simulink model "momentumBasedYoga"  (Simulink 9.0)
settings: Solver=FixedStepDiscrete  StartTime=0.0  StopTime="Config.SIMULATION_TIME "  FixedStep=Config.T_STEP  RelTol=1e-3  EnableMultiTasking=on
InitFcn:
  | cd(fileparts(which(bdroot)));
  | initMomentumBasedYoga;
StopFcn:
  | cd(fileparts(which(bdroot)));
  | stopMomentumBasedYoga;
undefined symbols (not defined in the file or in its folder): bVectorConstraints, Config, ConstraintsMatrix, Gain, Reg, ROBOT_DOF, ROBOT_DOF_FOR_SIMULINK, Sat, Sm
libraries: WBToolboxLibrary x80, simulink x4
(part 2 of 2)

== system momentumBasedYoga/Robot State and References/State Machine Yoga/Compute base to fixed link transform ==
  s : Inport
  inertial : Inport  Port=2
  Constant7 : Constant  Value=eye(4)
  "Floating Base to Fixed Link Transform (Left Foot) " : Subsystem
  Floating Base to Fixed Link Transform (Right Foot) : Subsystem
  LFoot to World Transform with Fixed Base : WBToolboxLibrary/wholeBodyModel/Kinematics/Forward Kinematics  frameName=Frames.LEFT_FOOT
      settings: SourceProductName=Whole Body Toolbox
  RFoot to World Transform with Fixed Base : WBToolboxLibrary/wholeBodyModel/Kinematics/Forward Kinematics  frameName=Frames.RIGHT_FOOT
      settings: SourceProductName=Whole Body Toolbox
  fixed_LFoot_H_b : Outport
  fixed_RFoot_H_b : Outport  Port=2
  wires:
  Constant7/1 -> RFoot to World Transform with Fixed Base/1, LFoot to World Transform with Fixed Base/1
  s/1 -> "Floating Base to Fixed Link Transform (Left Foot) "/1(s), Floating Base to Fixed Link Transform (Right Foot)/1(s), LFoot to World Transform with Fixed Base/2, RFoot to World Transform with Fixed Base/2
  "Floating Base to Fixed Link Transform (Left Foot) "/1(fixed_link_H_b) -> fixed_LFoot_H_b/1
  Floating Base to Fixed Link Transform (Right Foot)/1(fixed_link_H_b) -> fixed_RFoot_H_b/1
  RFoot to World Transform with Fixed Base/1 -> Floating Base to Fixed Link Transform (Right Foot)/3(w_H_fixed_link)
  LFoot to World Transform with Fixed Base/1 -> "Floating Base to Fixed Link Transform (Left Foot) "/3(w_H_fixed_link)
  inertial/1 -> "Floating Base to Fixed Link Transform (Left Foot) "/2(inertial), Floating Base to Fixed Link Transform (Right Foot)/2(inertial)

== system momentumBasedYoga/Robot State and References/State Machine Yoga/xCom ==
  w_H_b : Inport
  s : Inport  Port=2
  CoM : WBToolboxLibrary/wholeBodyModel/Kinematics/Forward Kinematics  frameName=Frames.COM
      settings: SourceProductName=Whole Body Toolbox
  "CoM6D ->  CoMXYZ2" : Selector  NumberOfDimensions=2  InputPortWidth=7  IndexOptions=Index vector (dialog),Index vector (dialog)  Indices=[1 2 3],[4]  OutputSizes=1,1
  x_CoM : Outport
  wires:
  s/1 -> CoM/2
  "CoM6D ->  CoMXYZ2"/1 -> x_CoM/1
  CoM/1 -> "CoM6D ->  CoMXYZ2"/1
  w_H_b/1 -> CoM/1

== system momentumBasedYoga/Robot State and References/State Machine Yoga/xCom1 ==
  w_H_b : Inport
  s : Inport  Port=2
  CoM : WBToolboxLibrary/wholeBodyModel/Kinematics/Forward Kinematics  frameName=Frames.COM
      settings: SourceProductName=Whole Body Toolbox
  "CoM6D ->  CoMXYZ2" : Selector  NumberOfDimensions=2  InputPortWidth=7  IndexOptions=Index vector (dialog),Index vector (dialog)  Indices=[1 2 3],[4]  OutputSizes=1,1
  x_CoM : Outport
  wires:
  s/1 -> CoM/2
  "CoM6D ->  CoMXYZ2"/1 -> x_CoM/1
  CoM/1 -> "CoM6D ->  CoMXYZ2"/1
  w_H_b/1 -> CoM/1

== system momentumBasedYoga/Balancing Controller QP/Approximate Momentum Integral/Compute base to fixed link transform/Floating Base to Fixed Link Transform (Left Foot)  ==
  s : Inport
  inertial : Inport  Port=2
  w_H_fixed_link : Inport  Port=3
  Constant : Constant  Value=eye(4)
  Imu to World Transform : WBToolboxLibrary/wholeBodyModel/Kinematics/Forward Kinematics  frameName=Frames.IMU
      settings: SourceProductName=Whole Body Toolbox
  Inv\* : Product  Inputs=/*  Multiplication=Matrix(*)
  "Inv\\*  " : Product  Inputs=/  Multiplication=Matrix(*)
  Neck Position : WBToolboxLibrary/Utilities/Yarp Read  portName=Ports.NECK_POS  signalSize=6  timeout=0.5  blocking=off  timestamp=off  autoconnect=on  errorOnConnection=off
      settings: SourceProductName=Whole Body Toolbox
  Neck Transform : Subsystem
  Switch6 : Switch  Criteria=u2 > Threshold
  USE_IMU4EST_BASE : Constant  Value=Config.USE_IMU4EST_BASE
  fromImuToHomogeousTransformFCN : MATLAB Function  TreatAsAtomicUnit=on
  holder 1 : WBToolboxLibrary/Utilities/holder 
      settings: SourceProductName=Whole Body Toolbox
  holder 2 : WBToolboxLibrary/Utilities/holder 
      settings: SourceProductName=Whole Body Toolbox
  fixed_link_H_b : Outport
  wires:
  Switch6/1 -> fixed_link_H_b/1
  "Inv\\*  "/1 -> fromImuToHomogeousTransformFCN/3(link_H_base), Switch6/3  "link_H_root"
  USE_IMU4EST_BASE/1 -> Switch6/2
  Inv\*/1 -> fromImuToHomogeousTransformFCN/1(imu_H_link), holder 1/1  "imu_H_link"
  holder 2/1 -> fromImuToHomogeousTransformFCN/4(inertial_0)
  Imu to World Transform/1 -> Inv\*/1
  holder 1/1 -> fromImuToHomogeousTransformFCN/2(imu_H_link_0)
  s/1 -> Imu to World Transform/2
  fromImuToHomogeousTransformFCN/1(w_H_b) -> Switch6/1
  inertial/1 -> holder 2/1, fromImuToHomogeousTransformFCN/5(inertial)
  Neck Position/1 -> Neck Transform/1(neck_port)
  Neck Transform/1(neck_pos) -> fromImuToHomogeousTransformFCN/6(neck_pos)
  w_H_fixed_link/1 -> "Inv\\*  "/1, Inv\*/2
  Constant/1 -> Imu to World Transform/1

== system momentumBasedYoga/Balancing Controller QP/Approximate Momentum Integral/Compute base to fixed link transform/Floating Base to Fixed Link Transform (Right Foot) ==
  s : Inport
  inertial : Inport  Port=2
  w_H_fixed_link : Inport  Port=3
  Constant : Constant  Value=eye(4)
  Imu to World Transform : WBToolboxLibrary/wholeBodyModel/Kinematics/Forward Kinematics  frameName=Frames.IMU
      settings: SourceProductName=Whole Body Toolbox
  Inv\* : Product  Inputs=/*  Multiplication=Matrix(*)
  "Inv\\*  " : Product  Inputs=/  Multiplication=Matrix(*)
  Neck Position : WBToolboxLibrary/Utilities/Yarp Read  portName=Ports.NECK_POS  signalSize=6  timeout=0.5  blocking=off  timestamp=off  autoconnect=on  errorOnConnection=off
      settings: SourceProductName=Whole Body Toolbox
  Neck Transform : Subsystem
  Switch6 : Switch  Criteria=u2 > Threshold
  USE_IMU4EST_BASE : Constant  Value=Config.USE_IMU4EST_BASE
  fromImuToHomogeousTransformFCN : MATLAB Function  TreatAsAtomicUnit=on
  holder 1 : WBToolboxLibrary/Utilities/holder 
      settings: SourceProductName=Whole Body Toolbox
  holder 2 : WBToolboxLibrary/Utilities/holder 
      settings: SourceProductName=Whole Body Toolbox
  fixed_link_H_b : Outport
  wires:
  Switch6/1 -> fixed_link_H_b/1
  "Inv\\*  "/1 -> fromImuToHomogeousTransformFCN/3(link_H_base), Switch6/3  "link_H_root"
  USE_IMU4EST_BASE/1 -> Switch6/2
  Inv\*/1 -> fromImuToHomogeousTransformFCN/1(imu_H_link), holder 1/1  "imu_H_link"
  holder 2/1 -> fromImuToHomogeousTransformFCN/4(inertial_0)
  Imu to World Transform/1 -> Inv\*/1
  holder 1/1 -> fromImuToHomogeousTransformFCN/2(imu_H_link_0)
  s/1 -> Imu to World Transform/2
  fromImuToHomogeousTransformFCN/1(w_H_b) -> Switch6/1
  inertial/1 -> holder 2/1, fromImuToHomogeousTransformFCN/5(inertial)
  Neck Position/1 -> Neck Transform/1(neck_port)
  Neck Transform/1(neck_pos) -> fromImuToHomogeousTransformFCN/6(neck_pos)
  w_H_fixed_link/1 -> "Inv\\*  "/1, Inv\*/2
  Constant/1 -> Imu to World Transform/1

== system momentumBasedYoga/Robot State and References/Internal Coordinator/Base to Fixed Link/Fixed Link to World Transform ==
  s : Inport
  Constant1 : Constant  Value=Config.LEFT_RIGHT_FOOT_IN_CONTACT(1)
  Constant7 : Constant  Value=eye(4)
  LFoot to World Transform with Fixed Base = World : WBToolboxLibrary/wholeBodyModel/Kinematics/Forward Kinematics  frameName=Frames.LEFT_FOOT
      settings: SourceProductName=Whole Body Toolbox
  RFoot to World Transform with Fixed Base = World : WBToolboxLibrary/wholeBodyModel/Kinematics/Forward Kinematics  frameName=Frames.RIGHT_FOOT
      settings: SourceProductName=Whole Body Toolbox
  Switch : Switch  Criteria=u2 > Threshold
  w_H_fixed_link : Outport
  wires:
  s/1 -> LFoot to World Transform with Fixed Base = World/2, RFoot to World Transform with Fixed Base = World/2
  Constant7/1 -> RFoot to World Transform with Fixed Base = World/1, LFoot to World Transform with Fixed Base = World/1
  Switch/1 -> w_H_fixed_link/1
  LFoot to World Transform with Fixed Base = World/1 -> Switch/1
  RFoot to World Transform with Fixed Base = World/1 -> Switch/3
  Constant1/1 -> Switch/2

== system momentumBasedYoga/Robot State and References/Internal Coordinator/Base to Fixed Link/Floating Base to Fixed Link Transform  ==
  s : Inport
  inertial : Inport  Port=2
  w_H_fixed_link : Inport  Port=3
  Constant : Constant  Value=eye(4)
  Imu to World Transform : WBToolboxLibrary/wholeBodyModel/Kinematics/Forward Kinematics  frameName=Frames.IMU
      settings: SourceProductName=Whole Body Toolbox
  Inv\* : Product  Inputs=/*  Multiplication=Matrix(*)
  "Inv\\*  " : Product  Inputs=/  Multiplication=Matrix(*)
  Neck Position : WBToolboxLibrary/Utilities/Yarp Read  portName=Ports.NECK_POS  signalSize=6  timeout=0.5  blocking=off  timestamp=off  autoconnect=on  errorOnConnection=off
      settings: SourceProductName=Whole Body Toolbox
  Neck Transform : Subsystem
  Switch6 : Switch  Criteria=u2 > Threshold
  USE_IMU4EST_BASE : Constant  Value=Config.USE_IMU4EST_BASE
  fromImuToHomogeousTransformFCN : MATLAB Function  TreatAsAtomicUnit=on
  holder 1 : WBToolboxLibrary/Utilities/holder 
      settings: SourceProductName=Whole Body Toolbox
  holder 2 : WBToolboxLibrary/Utilities/holder 
      settings: SourceProductName=Whole Body Toolbox
  fixed_link_H_b : Outport
  wires:
  Switch6/1 -> fixed_link_H_b/1
  "Inv\\*  "/1 -> fromImuToHomogeousTransformFCN/3(link_H_base), Switch6/3  "link_H_root"
  USE_IMU4EST_BASE/1 -> Switch6/2
  Inv\*/1 -> fromImuToHomogeousTransformFCN/1(imu_H_link), holder 1/1  "imu_H_link"
  holder 2/1 -> fromImuToHomogeousTransformFCN/4(inertial_0)
  Imu to World Transform/1 -> Inv\*/1
  holder 1/1 -> fromImuToHomogeousTransformFCN/2(imu_H_link_0)
  s/1 -> Imu to World Transform/2
  fromImuToHomogeousTransformFCN/1(w_H_b) -> Switch6/1
  inertial/1 -> holder 2/1, fromImuToHomogeousTransformFCN/5(inertial)
  Neck Position/1 -> Neck Transform/1(neck_port)
  Neck Transform/1(neck_pos) -> fromImuToHomogeousTransformFCN/6(neck_pos)
  w_H_fixed_link/1 -> "Inv\\*  "/1, Inv\*/2
  Constant/1 -> Imu to World Transform/1

== system momentumBasedYoga/Robot State and References/Internal Coordinator/Compute State Velocity/Feet Jacobians ==
  s : Inport
  w_H_b : Inport  Port=2
  Jacobian LFoot : WBToolboxLibrary/wholeBodyModel/Jacobians/Jacobian  frameName=Frames.LEFT_FOOT
      settings: SourceProductName=Whole Body Toolbox
  Jacobian RFoot : WBToolboxLibrary/wholeBodyModel/Jacobians/Jacobian  frameName=Frames.RIGHT_FOOT
      settings: SourceProductName=Whole Body Toolbox
  J_LFoot : Outport
  J_RFoot : Outport  Port=2
  wires:
  Jacobian LFoot/1 -> J_LFoot/1
  Jacobian RFoot/1 -> J_RFoot/1
  w_H_b/1 -> Jacobian RFoot/1, Jacobian LFoot/1
  s/1 -> Jacobian LFoot/2, Jacobian RFoot/2

== system momentumBasedYoga/Robot State and References/State Machine Yoga/Compute State Velocity/Feet Jacobians ==
  s : Inport
  w_H_b : Inport  Port=2
  Jacobian LFoot : WBToolboxLibrary/wholeBodyModel/Jacobians/Jacobian  frameName=Frames.LEFT_FOOT
      settings: SourceProductName=Whole Body Toolbox
  Jacobian RFoot : WBToolboxLibrary/wholeBodyModel/Jacobians/Jacobian  frameName=Frames.RIGHT_FOOT
      settings: SourceProductName=Whole Body Toolbox
  J_LFoot : Outport
  J_RFoot : Outport  Port=2
  wires:
  Jacobian LFoot/1 -> J_LFoot/1
  Jacobian RFoot/1 -> J_RFoot/1
  w_H_b/1 -> Jacobian RFoot/1, Jacobian LFoot/1
  s/1 -> Jacobian LFoot/2, Jacobian RFoot/2

== system momentumBasedYoga/Robot State and References/State Machine Yoga/Compute base to fixed link transform/Floating Base to Fixed Link Transform (Left Foot)  ==
  s : Inport
  inertial : Inport  Port=2
  w_H_fixed_link : Inport  Port=3
  Constant : Constant  Value=eye(4)
  Imu to World Transform : WBToolboxLibrary/wholeBodyModel/Kinematics/Forward Kinematics  frameName=Frames.IMU
      settings: SourceProductName=Whole Body Toolbox
  Inv\* : Product  Inputs=/*  Multiplication=Matrix(*)
  "Inv\\*  " : Product  Inputs=/  Multiplication=Matrix(*)
  Neck Position : WBToolboxLibrary/Utilities/Yarp Read  portName=Ports.NECK_POS  signalSize=6  timeout=0.5  blocking=off  timestamp=off  autoconnect=on  errorOnConnection=off
      settings: SourceProductName=Whole Body Toolbox
  Neck Transform : Subsystem
  Switch6 : Switch  Criteria=u2 > Threshold
  USE_IMU4EST_BASE : Constant  Value=Config.USE_IMU4EST_BASE
  fromImuToHomogeousTransformFCN : MATLAB Function  TreatAsAtomicUnit=on
  holder 1 : WBToolboxLibrary/Utilities/holder 
      settings: SourceProductName=Whole Body Toolbox
  holder 2 : WBToolboxLibrary/Utilities/holder 
      settings: SourceProductName=Whole Body Toolbox
  fixed_link_H_b : Outport
  wires:
  Switch6/1 -> fixed_link_H_b/1
  "Inv\\*  "/1 -> fromImuToHomogeousTransformFCN/3(link_H_base), Switch6/3  "link_H_root"
  USE_IMU4EST_BASE/1 -> Switch6/2
  Inv\*/1 -> fromImuToHomogeousTransformFCN/1(imu_H_link), holder 1/1  "imu_H_link"
  holder 2/1 -> fromImuToHomogeousTransformFCN/4(inertial_0)
  Imu to World Transform/1 -> Inv\*/1
  holder 1/1 -> fromImuToHomogeousTransformFCN/2(imu_H_link_0)
  s/1 -> Imu to World Transform/2
  fromImuToHomogeousTransformFCN/1(w_H_b) -> Switch6/1
  inertial/1 -> holder 2/1, fromImuToHomogeousTransformFCN/5(inertial)
  Neck Position/1 -> Neck Transform/1(neck_port)
  Neck Transform/1(neck_pos) -> fromImuToHomogeousTransformFCN/6(neck_pos)
  w_H_fixed_link/1 -> "Inv\\*  "/1, Inv\*/2
  Constant/1 -> Imu to World Transform/1

== system momentumBasedYoga/Robot State and References/State Machine Yoga/Compute base to fixed link transform/Floating Base to Fixed Link Transform (Right Foot) ==
  s : Inport
  inertial : Inport  Port=2
  w_H_fixed_link : Inport  Port=3
  Constant : Constant  Value=eye(4)
  Imu to World Transform : WBToolboxLibrary/wholeBodyModel/Kinematics/Forward Kinematics  frameName=Frames.IMU
      settings: SourceProductName=Whole Body Toolbox
  Inv\* : Product  Inputs=/*  Multiplication=Matrix(*)
  "Inv\\*  " : Product  Inputs=/  Multiplication=Matrix(*)
  Neck Position : WBToolboxLibrary/Utilities/Yarp Read  portName=Ports.NECK_POS  signalSize=6  timeout=0.5  blocking=off  timestamp=off  autoconnect=on  errorOnConnection=off
      settings: SourceProductName=Whole Body Toolbox
  Neck Transform : Subsystem
  Switch6 : Switch  Criteria=u2 > Threshold
  USE_IMU4EST_BASE : Constant  Value=Config.USE_IMU4EST_BASE
  fromImuToHomogeousTransformFCN : MATLAB Function  TreatAsAtomicUnit=on
  holder 1 : WBToolboxLibrary/Utilities/holder 
      settings: SourceProductName=Whole Body Toolbox
  holder 2 : WBToolboxLibrary/Utilities/holder 
      settings: SourceProductName=Whole Body Toolbox
  fixed_link_H_b : Outport
  wires:
  Switch6/1 -> fixed_link_H_b/1
  "Inv\\*  "/1 -> fromImuToHomogeousTransformFCN/3(link_H_base), Switch6/3  "link_H_root"
  USE_IMU4EST_BASE/1 -> Switch6/2
  Inv\*/1 -> fromImuToHomogeousTransformFCN/1(imu_H_link), holder 1/1  "imu_H_link"
  holder 2/1 -> fromImuToHomogeousTransformFCN/4(inertial_0)
  Imu to World Transform/1 -> Inv\*/1
  holder 1/1 -> fromImuToHomogeousTransformFCN/2(imu_H_link_0)
  s/1 -> Imu to World Transform/2
  fromImuToHomogeousTransformFCN/1(w_H_b) -> Switch6/1
  inertial/1 -> holder 2/1, fromImuToHomogeousTransformFCN/5(inertial)
  Neck Position/1 -> Neck Transform/1(neck_port)
  Neck Transform/1(neck_pos) -> fromImuToHomogeousTransformFCN/6(neck_pos)
  w_H_fixed_link/1 -> "Inv\\*  "/1, Inv\*/2
  Constant/1 -> Imu to World Transform/1

== system momentumBasedYoga/Balancing Controller QP/Approximate Momentum Integral/Compute base to fixed link transform/Floating Base to Fixed Link Transform (Left Foot) /Neck Transform ==
  neck_port : Inport
  Constant : Constant  Value=zeros(3,1)
  Gain : Gain  Gain=pi/180
  Selector1 : Selector  InputPortWidth=6  IndexOptions=Index vector (dialog)  Indices=[1:3]  OutputSizes=1
  Switch : Switch  Criteria=u2 > Threshold
  USE_IMU4EST_BASE1 : Constant  Value=Config.CORRECT_NECK_IMU
  neck_pos : Outport
  wires:
  neck_port/1 -> Gain/1
  USE_IMU4EST_BASE1/1 -> Switch/2
  Switch/1 -> neck_pos/1
  Gain/1 -> Selector1/1
  Constant/1 -> Switch/3
  Selector1/1 -> Switch/1  "neck pos"

== system momentumBasedYoga/Balancing Controller QP/Approximate Momentum Integral/Compute base to fixed link transform/Floating Base to Fixed Link Transform (Right Foot)/Neck Transform ==
  neck_port : Inport
  Constant : Constant  Value=zeros(3,1)
  Gain : Gain  Gain=pi/180
  Selector1 : Selector  InputPortWidth=6  IndexOptions=Index vector (dialog)  Indices=[1:3]  OutputSizes=1
  Switch : Switch  Criteria=u2 > Threshold
  USE_IMU4EST_BASE1 : Constant  Value=Config.CORRECT_NECK_IMU
  neck_pos : Outport
  wires:
  neck_port/1 -> Gain/1
  USE_IMU4EST_BASE1/1 -> Switch/2
  Switch/1 -> neck_pos/1
  Gain/1 -> Selector1/1
  Constant/1 -> Switch/3
  Selector1/1 -> Switch/1  "neck pos"

== system momentumBasedYoga/Robot State and References/Internal Coordinator/Base to Fixed Link/Floating Base to Fixed Link Transform /Neck Transform ==
  neck_port : Inport
  Constant : Constant  Value=zeros(3,1)
  Gain : Gain  Gain=pi/180
  Selector1 : Selector  InputPortWidth=6  IndexOptions=Index vector (dialog)  Indices=[1:3]  OutputSizes=1
  Switch : Switch  Criteria=u2 > Threshold
  USE_IMU4EST_BASE1 : Constant  Value=Config.CORRECT_NECK_IMU
  neck_pos : Outport
  wires:
  neck_port/1 -> Gain/1
  USE_IMU4EST_BASE1/1 -> Switch/2
  Switch/1 -> neck_pos/1
  Gain/1 -> Selector1/1
  Constant/1 -> Switch/3
  Selector1/1 -> Switch/1  "neck pos"

== system momentumBasedYoga/Robot State and References/State Machine Yoga/Compute base to fixed link transform/Floating Base to Fixed Link Transform (Left Foot) /Neck Transform ==
  neck_port : Inport
  Constant : Constant  Value=zeros(3,1)
  Gain : Gain  Gain=pi/180
  Selector1 : Selector  InputPortWidth=6  IndexOptions=Index vector (dialog)  Indices=[1:3]  OutputSizes=1
  Switch : Switch  Criteria=u2 > Threshold
  USE_IMU4EST_BASE1 : Constant  Value=Config.CORRECT_NECK_IMU
  neck_pos : Outport
  wires:
  neck_port/1 -> Gain/1
  USE_IMU4EST_BASE1/1 -> Switch/2
  Switch/1 -> neck_pos/1
  Gain/1 -> Selector1/1
  Constant/1 -> Switch/3
  Selector1/1 -> Switch/1  "neck pos"

== system momentumBasedYoga/Robot State and References/State Machine Yoga/Compute base to fixed link transform/Floating Base to Fixed Link Transform (Right Foot)/Neck Transform ==
  neck_port : Inport
  Constant : Constant  Value=zeros(3,1)
  Gain : Gain  Gain=pi/180
  Selector1 : Selector  InputPortWidth=6  IndexOptions=Index vector (dialog)  Indices=[1:3]  OutputSizes=1
  Switch : Switch  Criteria=u2 > Threshold
  USE_IMU4EST_BASE1 : Constant  Value=Config.CORRECT_NECK_IMU
  neck_pos : Outport
  wires:
  neck_port/1 -> Gain/1
  USE_IMU4EST_BASE1/1 -> Switch/2
  Switch/1 -> neck_pos/1
  Gain/1 -> Selector1/1
  Constant/1 -> Switch/3
  Selector1/1 -> Switch/1  "neck pos"

== matlab function Balancing Controller QP/Approximate Momentum Integral/Compute base to fixed link transform/Floating Base to Fixed Link Transform (Left Foot) /fromImuToHomogeousTransformFCN ==
  data: imu_H_link input double; imu_H_link_0 input double; link_H_base input double; inertial_0 input double; inertial input double; neck_pos input double; w_H_b output double; Config parameter double
function w_H_b = worldToBaseTransformWithIMUFCN(imu_H_link,imu_H_link_0,link_H_base,inertial_0,inertial,neck_pos,Config)

    w_H_b = worldToBaseTransformWithIMU(imu_H_link,imu_H_link_0,link_H_base,inertial_0,inertial,neck_pos,Config);

end

== matlab function Robot State and References/Internal Coordinator/Base to Fixed Link/Floating Base to Fixed Link Transform /fromImuToHomogeousTransformFCN ==
  data: imu_H_link input double; imu_H_link_0 input double; link_H_base input double; inertial_0 input double; inertial input double; neck_pos input double; w_H_b output double; Config parameter double
function w_H_b = worldToBaseTransformWithIMUFCN(imu_H_link,imu_H_link_0,link_H_base,inertial_0,inertial,neck_pos,Config)

    w_H_b = worldToBaseTransformWithIMU(imu_H_link,imu_H_link_0,link_H_base,inertial_0,inertial,neck_pos,Config);

end

== matlab function Robot State and References/State Machine Yoga/Compute base to fixed link transform/Floating Base to Fixed Link Transform (Left Foot) /fromImuToHomogeousTransformFCN ==
  data: imu_H_link input double; imu_H_link_0 input double; link_H_base input double; inertial_0 input double; inertial input double; neck_pos input double; w_H_b output double; Config parameter double
function w_H_b = worldToBaseTransformWithIMUFCN(imu_H_link,imu_H_link_0,link_H_base,inertial_0,inertial,neck_pos,Config)

    w_H_b = worldToBaseTransformWithIMU(imu_H_link,imu_H_link_0,link_H_base,inertial_0,inertial,neck_pos,Config);

end

== matlab function Balancing Controller QP/Approximate Momentum Integral/Compute base to fixed link transform/Floating Base to Fixed Link Transform (Right Foot)/fromImuToHomogeousTransformFCN ==
  data: imu_H_link input double; imu_H_link_0 input double; link_H_base input double; inertial_0 input double; inertial input double; neck_pos input double; w_H_b output double; Config parameter double
function w_H_b = worldToBaseTransformWithIMUFCN(imu_H_link,imu_H_link_0,link_H_base,inertial_0,inertial,neck_pos,Config)

    w_H_b = worldToBaseTransformWithIMU(imu_H_link,imu_H_link_0,link_H_base,inertial_0,inertial,neck_pos,Config);

end

== matlab function Robot State and References/Internal Coordinator/Compute State Velocity/Compute Base Velocity ==
  data: J_LeftFoot input double; J_RightFoot input double; feet_in_contact input double; nu_b output double; sDot input double; Reg parameter double
function nu_b = computeBaseVelocityFCN(J_LeftFoot, J_RightFoot, feet_in_contact, sDot, Reg)

    nu_b = computeBaseVelocity(J_LeftFoot, J_RightFoot, feet_in_contact, sDot, Reg);
end

== matlab function Dynamics and Kinematics/Dynamics Variables/Add Motors Reflected Inertia/Add Motor Reflected Inertia ==
  data: M input double; M_with_inertia output double; Config parameter double
function M_with_inertia = addMotorsInertiaFCN(M,Config)

    M_with_inertia = addMotorsInertia(M,Config);

end

== matlab function Robot State and References/State Machine Yoga/Compute State Velocity/Compute Base Velocity ==
  data: J_LeftFoot input double; J_RightFoot input double; feet_in_contact input double; nu_b output double; sDot input double; Reg parameter double
function nu_b = computeBaseVelocityFCN(J_LeftFoot, J_RightFoot, feet_in_contact, sDot, Reg)

    nu_b = computeBaseVelocity(J_LeftFoot, J_RightFoot, feet_in_contact, sDot, Reg);
end

== matlab function Robot State and References/State Machine Yoga/Compute base to fixed link transform/Floating Base to Fixed Link Transform (Right Foot)/fromImuToHomogeousTransformFCN ==
  data: imu_H_link input double; imu_H_link_0 input double; link_H_base input double; inertial_0 input double; inertial input double; neck_pos input double; w_H_b output double; Config parameter double
function w_H_b = worldToBaseTransformWithIMUFCN(imu_H_link,imu_H_link_0,link_H_base,inertial_0,inertial,neck_pos,Config)

    w_H_b = worldToBaseTransformWithIMU(imu_H_link,imu_H_link_0,link_H_base,inertial_0,inertial,neck_pos,Config);

end

== matlab function Balancing Controller QP/Compute Joint Torques/(transpose(T*Gamma))^{-1}*I_m*(T*Gamma)^{-1} ==
  data: reflectedInertia output double; Config parameter double
function reflectedInertia  = computeMotorsInertiaFCN(Config)

    [reflectedInertia] = computeMotorsInertia(Config);

end

== matlab function Robot State and References/Internal Coordinator/Reference Generator CoM ==
  data: pos_CoM_0 input double; t input double; references_CoM output double; Config parameter double
function references_CoM = referenceGeneratorCoMFCN(pos_CoM_0, t, Config)

    references_CoM = referenceGeneratorCoM(pos_CoM_0, t, Config);
end

== matlab function Robot State and References/State Machine Yoga/stateMachineYogaFCN ==
  data: wrench_rightFoot input double; wrench_leftFoot input double; w_H_b output double; CoM_des output double; s_des output double; feet_in_contact output double; CoM_0 input double; s_0 input double; l_sole_CoM input double; r_sole_CoM input double; s input double; t input double; l_sole_H_b input double; r_sole_H_b input double; Sm parameter double; Kp_joints output double; Kp_CoM output double; Kd_CoM output double; Gain parameter double; current_state output double; smoothingTime_CoM_joints output double
function [w_H_b, CoM_des, s_des, feet_in_contact, Kp_joints, Kp_CoM, Kd_CoM, current_state, smoothingTime_CoM_joints] = ...
          stateMachineYogaFCN(wrench_rightFoot, wrench_leftFoot, CoM_0, s_0, l_sole_CoM, r_sole_CoM, s, t, l_sole_H_b, r_sole_H_b, Sm, Gain)
 
    [w_H_b, CoM_des, s_des, feet_in_contact, Kp_joints, Kp_CoM, Kd_CoM, current_state, smoothingTime_CoM_joints] = ...
        stateMachineYoga(CoM_0, s_0, l_sole_CoM, r_sole_CoM, s, t, wrench_rightFoot, wrench_leftFoot, l_sole_H_b, r_sole_H_b, Sm, Gain); 
end

== matlab function Balancing Controller QP/Balancing Controller  ==
  data: tau_model output double; Sigma output double; Null_A output double; f_LDot_des output double; HessianMatrix_QP1Foot output double; gradient_QP1Foot output double; ConstraintsMatrix_QP1Foot output double; bVectorConstraints_Qp1Foot output double; HessianMatrix_QP2Feet output double; gradient_QP2Feet output double; ConstraintsMatrix_QP2Feet output double; bVectorConstraints_Qp2Feet output double; feet_in_contact input double; ROBOT_DOF_FOR_SIMULINK input double; ConstraintsMatrix input double; bVectorConstraints input double; s input double; s_des input double; nu input double; M input double; h input double; L input double; intL input double; w_H_l_sole input double; w_H_r_sole input double; J_l_sole input double; J_r_sole input double; JDot_l_sole_nu input double; JDot_r_sole_nu input double; x_CoM input double; J_CoM input double; desired_x_xDot_xDDot_CoM input double; Kp_CoM input double; Kd_CoM input double; Kp_joints input double; CoM_error output double; Gain parameter double; Reg parameter double
function [tau_model, Sigma, Null_A, f_LDot_des, ...
          HessianMatrix_QP1Foot, gradient_QP1Foot, ConstraintsMatrix_QP1Foot, bVectorConstraints_Qp1Foot, ...
          HessianMatrix_QP2Feet, gradient_QP2Feet, ConstraintsMatrix_QP2Feet, bVectorConstraints_Qp2Feet, ...
          CoM_error] = ...
              balancingControllerYogaFCN(feet_in_contact, ROBOT_DOF_FOR_SIMULINK, ConstraintsMatrix, bVectorConstraints, ...
                  s, s_des, nu, M, h, L, intL, w_H_l_sole, w_H_r_sole, J_l_sole, J_r_sole, JDot_l_sole_nu, JDot_r_sole_nu, x_CoM, J_CoM, ...
                  desired_x_xDot_xDDot_CoM, Kp_CoM, Kd_CoM, Kp_joints, Gain, Reg)
          
    [tau_model, Sigma, Null_A, f_LDot_des, ...
     HessianMatrix_QP1Foot, gradient_QP1Foot, ConstraintsMatrix_QP1Foot, bVectorConstraints_Qp1Foot, ...
     HessianMatrix_QP2Feet, gradient_QP2Feet, ConstraintsMatrix_QP2Feet, bVectorConstraints_Qp2Feet, ...
     CoM_error] = ...
         balancingControllerYoga(feet_in_contact, ROBOT_DOF_FOR_SIMULINK, ConstraintsMatrix, bVectorConstraints, ...
                                 s, s_des, nu, M, h, L, intL, w_H_l_sole, w_H_r_sole, J_l_sole, J_r_sole, JDot_l_sole_nu, JDot_r_sole_nu, x_CoM, J_CoM, ...
                                 desired_x_xDot_xDDot_CoM, Kp_CoM, Kd_CoM, Kp_joints, Reg, Gain);
end

== matlab function emergency stop: joint limits/MATLAB Function ==
  data: umin input double; umax input double; u input double; inRange output double; tol input double
function inRange = checkRangeFCN(umin, umax, u, tol)

     inRange = checkRange(umin, umax, u, tol);
end

== matlab function Balancing Controller QP/Approximate Momentum Integral/choose base to world transform ==
  data: state input double; booleanState output double
function booleanState = footOnGround(state)

    % output: a boolean variable whose value is 1 if the foot on ground is left
    % foot, and 0 if the foot on ground is the right foot. If both feet are on
    % ground, the variable is setted to 1.

    % states in which right foot is on ground: 9,10,11,12
    booleanState = 1;

    if state == 9 || state == 10 || state == 11 || state == 12

        booleanState = 0;
    end
end

== matlab function Balancing Controller QP/Approximate Momentum Integral/References for L ==
  data: s_err input double; JL input double; JR input double; nu_b_equivalent output double; Reg parameter double; activeFeetConstraints input double
function nu_b_equivalent = generateReferencesForH_FCN(s_err, JL, JR, Reg, activeFeetConstraints)

    if activeFeetConstraints(1) == 1
    
        pinvJb          = (JL(:,1:6)'*JL(:,1:6) + Reg.pinvDamp_nu_b*eye(6))\JL(:,1:6)';
        nu_b_equivalent = -pinvJb*JL(:,7:end)*s_err;
    else
    
        pinvJb          = (JR(:,1:6)'*JR(:,1:6) + Reg.pinvDamp_nu_b*eye(6))\JR(:,1:6)';
        nu_b_equivalent = -pinvJb*JR(:,7:end)*s_err;
    end
end
